simulink model "gm_parallel_8_min_cost_function"  (R2022a)
settings: Solver=FixedStepDiscrete  StartTime=0.0  StopTime=10.0  RelTol=1e-3
undefined symbols (not defined in the file or in its folder): f_c
libraries: hdlmdlgenlib x40
(part 2 of 2)

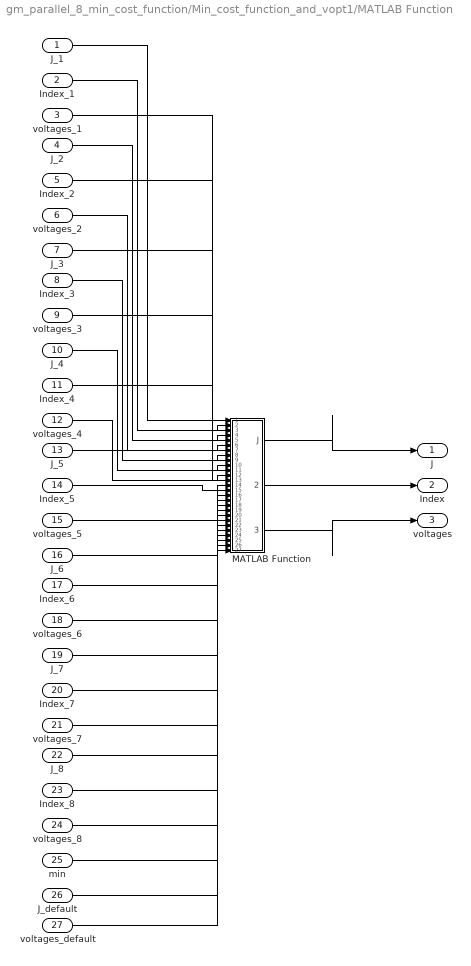
== system gm_parallel_8_min_cost_function/Min_cost_function_and_vopt1/MATLAB Function ==
  J_1 : Inport  OutDataTypeStr=fixdt(1, 20, 9)  PortDimensions=1  SampleTime=1e-08
  Index_1 : Inport  Port=2  OutDataTypeStr=int32  PortDimensions=1  SampleTime=1e-08
  voltages_1 : Inport  Port=3  OutDataTypeStr=fixdt(1, 24, 11)  PortDimensions=[4]  SampleTime=1e-08
  J_2 : Inport  Port=4  OutDataTypeStr=fixdt(1, 20, 9)  PortDimensions=1  SampleTime=1e-08
  Index_2 : Inport  Port=5  OutDataTypeStr=int32  PortDimensions=1  SampleTime=1e-08
  voltages_2 : Inport  Port=6  OutDataTypeStr=fixdt(1, 24, 11)  PortDimensions=[4]  SampleTime=1e-08
  J_3 : Inport  Port=7  OutDataTypeStr=fixdt(1, 20, 9)  PortDimensions=1  SampleTime=1e-08
  Index_3 : Inport  Port=8  OutDataTypeStr=int32  PortDimensions=1  SampleTime=1e-08
  voltages_3 : Inport  Port=9  OutDataTypeStr=fixdt(1, 24, 11)  PortDimensions=[4]  SampleTime=1e-08
  J_4 : Inport  Port=10  OutDataTypeStr=fixdt(1, 20, 9)  PortDimensions=1  SampleTime=1e-08
  Index_4 : Inport  Port=11  OutDataTypeStr=int32  PortDimensions=1  SampleTime=1e-08
  voltages_4 : Inport  Port=12  OutDataTypeStr=fixdt(1, 24, 11)  PortDimensions=[4]  SampleTime=1e-08
  J_5 : Inport  Port=13  OutDataTypeStr=fixdt(1, 20, 9)  PortDimensions=1  SampleTime=1e-08
  Index_5 : Inport  Port=14  OutDataTypeStr=int32  PortDimensions=1  SampleTime=1e-08
  voltages_5 : Inport  Port=15  OutDataTypeStr=fixdt(1, 24, 11)  PortDimensions=[4]  SampleTime=1e-08
  J_6 : Inport  Port=16  OutDataTypeStr=fixdt(1, 20, 9)  PortDimensions=1  SampleTime=1e-08
  Index_6 : Inport  Port=17  OutDataTypeStr=int32  PortDimensions=1  SampleTime=1e-08
  voltages_6 : Inport  Port=18  OutDataTypeStr=fixdt(1, 24, 11)  PortDimensions=[4]  SampleTime=1e-08
  J_7 : Inport  Port=19  OutDataTypeStr=fixdt(1, 20, 9)  PortDimensions=1  SampleTime=1e-08
  Index_7 : Inport  Port=20  OutDataTypeStr=int32  PortDimensions=1  SampleTime=1e-08
  voltages_7 : Inport  Port=21  OutDataTypeStr=fixdt(1, 24, 11)  PortDimensions=[4]  SampleTime=1e-08
  J_8 : Inport  Port=22  OutDataTypeStr=fixdt(1, 20, 9)  PortDimensions=1  SampleTime=1e-08
  Index_8 : Inport  Port=23  OutDataTypeStr=int32  PortDimensions=1  SampleTime=1e-08
  voltages_8 : Inport  Port=24  OutDataTypeStr=fixdt(1, 24, 11)  PortDimensions=[4]  SampleTime=1e-08
  min : Inport  Port=25  OutDataTypeStr=fixdt(1, 20, 9)  PortDimensions=1  SampleTime=1e-08
  J_default : Inport  Port=26  OutDataTypeStr=fixdt(1, 20, 9)  PortDimensions=1  SampleTime=1e-08
  voltages_default : Inport  Port=27  OutDataTypeStr=fixdt(1, 24, 11)  PortDimensions=[4]  SampleTime=1e-08
  MATLAB Function : MATLAB Function  TreatAsAtomicUnit=on  SystemSampleTime=1/100000000
  J : Outport  SampleTime=1e-08  VectorParamsAs1DForOutWhenUnconnected=off
  Index : Outport  Port=2  SampleTime=1e-08
  voltages : Outport  Port=3  SampleTime=1e-08
  wires:
  J_1/1 -> MATLAB Function/1(J_1)
  Index_1/1 -> MATLAB Function/2(Index_1)
  voltages_1/1 -> MATLAB Function/3(voltages_1)
  J_2/1 -> MATLAB Function/4(J_2)
  Index_2/1 -> MATLAB Function/5(Index_2)
  voltages_2/1 -> MATLAB Function/6(voltages_2)
  J_3/1 -> MATLAB Function/7(J_3)
  Index_3/1 -> MATLAB Function/8(Index_3)
  voltages_3/1 -> MATLAB Function/9(voltages_3)
  J_4/1 -> MATLAB Function/10(J_4)
  Index_4/1 -> MATLAB Function/11(Index_4)
  voltages_4/1 -> MATLAB Function/12(voltages_4)
  J_5/1 -> MATLAB Function/13(J_5)
  Index_5/1 -> MATLAB Function/14(Index_5)
  voltages_5/1 -> MATLAB Function/15(voltages_5)
  J_6/1 -> MATLAB Function/16(J_6)
  Index_6/1 -> MATLAB Function/17(Index_6)
  voltages_6/1 -> MATLAB Function/18(voltages_6)
  J_7/1 -> MATLAB Function/19(J_7)
  Index_7/1 -> MATLAB Function/20(Index_7)
  voltages_7/1 -> MATLAB Function/21(voltages_7)
  J_8/1 -> MATLAB Function/22(J_8)
  Index_8/1 -> MATLAB Function/23(Index_8)
  voltages_8/1 -> MATLAB Function/24(voltages_8)
  min/1 -> MATLAB Function/25(min)
  J_default/1 -> MATLAB Function/26(J_default)
  voltages_default/1 -> MATLAB Function/27(voltages_default)
  MATLAB Function/1(J) -> J/1
  MATLAB Function/2(Index) -> Index/1
  MATLAB Function/3(voltages) -> voltages/1

== system gm_parallel_8_min_cost_function/Min_cost_function_and_vopt1/Detect Rise Positive/Positive ==
  u : Inport  OutDataTypeStr=boolean  SampleTime=1e-08
  Compare : RelationalOperator  Operator=>  OutDataTypeStr=boolean  ZeroCross=off
  Constant : Constant  DisableCoverage=on  Value=0  OutDataTypeStr=Inherit: Inherit via back propagation  SampleTime=-1  PreserveConstantTs=on
  y : Outport  SampleTime=1e-08
  wires:
  u/1 -> Compare/1
  Compare/1 -> y/1
  Constant/1 -> Compare/2

== system gm_parallel_8_min_cost_function/Min_cost_function_and_vopt1/Detect Rise Positive1/Positive ==
  u : Inport  OutDataTypeStr=boolean  SampleTime=1e-08
  Compare : RelationalOperator  Operator=>  OutDataTypeStr=boolean  ZeroCross=off
  Constant : Constant  DisableCoverage=on  Value=0  OutDataTypeStr=Inherit: Inherit via back propagation  SampleTime=-1  PreserveConstantTs=on
  y : Outport  SampleTime=1e-08
  wires:
  u/1 -> Compare/1
  Compare/1 -> y/1
  Constant/1 -> Compare/2

== matlab function gm_parallel_8_min_cost_function/Min_cost_function_and_vopt1/MATLAB Function/MATLAB Function ==
  data: J_1 input; Index_1 input int32; J output; voltages_1 input; J_2 input; Index_2 input int32; voltages_2 input; J_3 input; Index_3 input int32; voltages_3 input; J_4 input; Index_4 input int32; voltages_4 input; J_5 input; Index_5 input int32; voltages_5 input; J_6 input; Index_6 input int32; voltages_6 input; J_7 input; Index_7 input int32; voltages_7 input; J_8 input; Index_8 input int32; voltages_8 input; Index output int32; voltages output; min input; J_default input; voltages_default input
function [J, Index, voltages] = fcn(J_1, Index_1, voltages_1, J_2, Index_2, voltages_2, J_3, Index_3, voltages_3, J_4, Index_4, voltages_4, J_5, Index_5, voltages_5, J_6, Index_6, voltages_6, ...
                                    J_7, Index_7, voltages_7, J_8, Index_8, voltages_8, min, J_default,voltages_default)



if J_1 == min
    Index = Index_1;
    voltages = voltages_1;
    J = J_1;
elseif J_2 == min
    Index = Index_2;
    voltages = voltages_2;
    J = J_2;
elseif J_3 == min
    Index = Index_3;
    voltages = voltages_3;
    J = J_3;
elseif J_4 == min
    Index = Index_4;
    voltages = voltages_4;
    J = J_4;
elseif J_5 == min
    Index = Index_5;
    voltages = voltages_5;
    J = J_5;
elseif J_6 == min
    Index = Index_6;
    voltages = voltages_6;
    J = J_6;
elseif J_7 == min
    Index = Index_7;
    voltages = voltages_7;
    J = J_7;
elseif J_8 == min
    Index = Index_8;
    voltages = voltages_8;
    J = J_8;
else 
    Index = int32(0);
    J = J_default;
    voltages = voltages_default;
end
